simulink model "eins_d"  (R2023a)
settings: Solver=VariableStepAuto  StartTime=0.0  StopTime=10.0  RelTol=1e-3
settings Model: Creator=alexa  LastModifiedBy=alexa

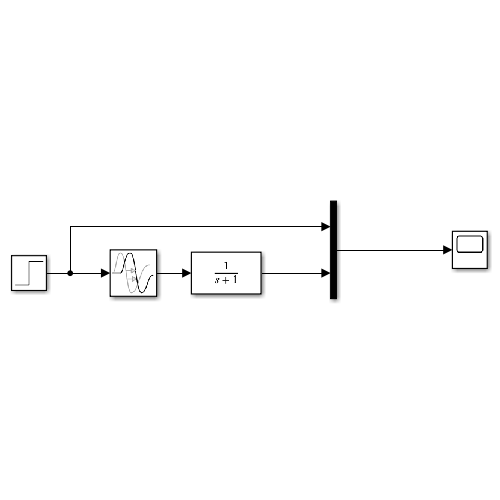
[thumbnail: Simulink's stored preview of the top-level diagram]
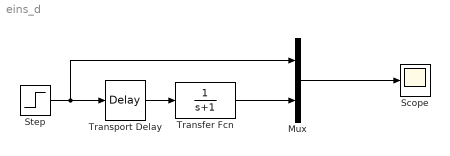
== system eins_d ==
  Mux : Mux  Inputs=2
  Scope : Scope
  Step : Step  SampleTime=0
  Transfer Fcn : TransferFcn  Denominator=[1 1]
  Transport Delay : TransportDelay
  wires:
  Step/1 -> Mux/1, Transport Delay/1
  Transfer Fcn/1 -> Mux/2
  Mux/1 -> Scope/1
  Transport Delay/1 -> Transfer Fcn/1
